simulink model "ThreeDOFsys"  (R2019a)
settings: Solver=ode3  StartTime=0.0  StopTime=120.0  FixedStep=.01  RelTol=1e-3  EnableMultiTasking=on
InitFcn:
  | % k1=25/1.5; k2=5/1.5; k3=30/1.5; k4=k3; c1=2.5; c2=.5; c3=3.5;
  | % m1=2.5; m2=2; m3=3;
  | F1 = 20; F2=0; F3=20;   % Case # 1
  | % F1 = 0; F2=0; F3=0;   % Case # 2
values from neighbouring files (symbols this model uses):
  c1 = 2.5    [MASS3.m]    (also in SMsysSIM.m = 2; three_MASS.m; two_DOF_sys_sim_ALL.m = 2)
  c2 = .5    (= 0.5)    [MASS3.m]    (also in SMsysSIM.m = 1; three_MASS.m; two_DOF_sys_sim_ALL.m = 1)
  c3 = 3.5    [MASS3.m]    (also in SMsysSIM.m = 3; three_MASS.m; two_DOF_sys_sim_ALL.m = 3)
  IC = [0;0;0;0;0;0]    [MASS3.m]    (also in three_MASS.m)
  k1 = 25    [MASS3.m]    (also in SMsysSIM.m = 90; three_MASS.m; two_DOF_sys_sim_ALL.m = 90)
  k2 = 5    [MASS3.m]    (also in SMsysSIM.m = 85; three_MASS.m; two_DOF_sys_sim_ALL.m = 85)
  k3 = 30    [MASS3.m]    (also in three_MASS.m)
  k4 = k3    (= 30)    [MASS3.m]    (also in three_MASS.m)
  m1 = 10    [DOUBLE_Pedulum_Linear_2.m]    (also in DOUBLE_Pedulum_Model_2.m; MASS3.m = 2.5; SMsysSIM.m = 5; three_MASS.m = 2.5)
  m2 = 10    [DOUBLE_Pedulum_Linear_2.m]    (also in DOUBLE_Pedulum_Model_2.m; MASS3.m = 2; SMsysSIM.m = 3; three_MASS.m = 2)
  m3 = 3    [MASS3.m]    (also in three_MASS.m)
settings Model: Creator=SLE  LastModifiedBy=sulaymon.eshkabilov
settings DataIOCC: LimitDataPoints=on  SaveFormat=Array  SignalLoggingSaveFormat=ModelDataLogs  ReturnWorkspaceOutputs=off
settings OptimizationCC: ExpressionDepthLimit=2147483647  LifeSpan=inf
settings DebuggingCC: UnderspecifiedInitializationDetection=Classic  MergeDetectMultiDrivingBlocksExec=none  SolverPrmCheckMsg=warning  FcnCallInpInsideContextMsg=warning  StateNameClashWarn=warning  SFUnexpectedBacktrackingDiag=warning  SFNoUnconditionalDefaultTransitionDiag=warning  SFExecutionAtInitializationDiag=none  ArithmeticOperatorsInVariantConditions=warning
settings HardwareCC: ProdBitPerPointer=32  ProdBitPerSizeT=32  ProdBitPerPtrDiffT=32  ProdLargestAtomicFloat=None  ProdIntDivRoundTo=Undefined  ProdEndianess=Unspecified  ProdWordSize=32  ProdHWDeviceType=32-bit Generic
settings ModelReferenceCC: PropagateSignalLabelsOutOfModel=off
settings SFSimCC: SimUseLocalCustomCode=off
settings RTWCC: GenCodeOnly=on  GenerateReport=on  TLCDebug=on  TLCAssert=on  RTWUseLocalCustomCode=off  RTWUseSimCustomCode=on  LaunchReport=on  TargetLang=C++
settings CodeAppCC: ForceParamTrailComments=on  StateflowObjectComments=on  UseSimReservedNames=on
settings GRTTargetCC: TargetLangStandard=C89/C90 (ANSI)  GeneratePreprocessorConditionals=Disable all  CombineOutputUpdateFcns=off  GRTInterface=on
settings ConfigComp: CovMetricSettings=dw  CovHtmlReporting=on  CovSaveCumulativeToWorkspaceVar=on  CovSaveSingleToWorkspaceVar=on  CovExternalEMLEnable=off

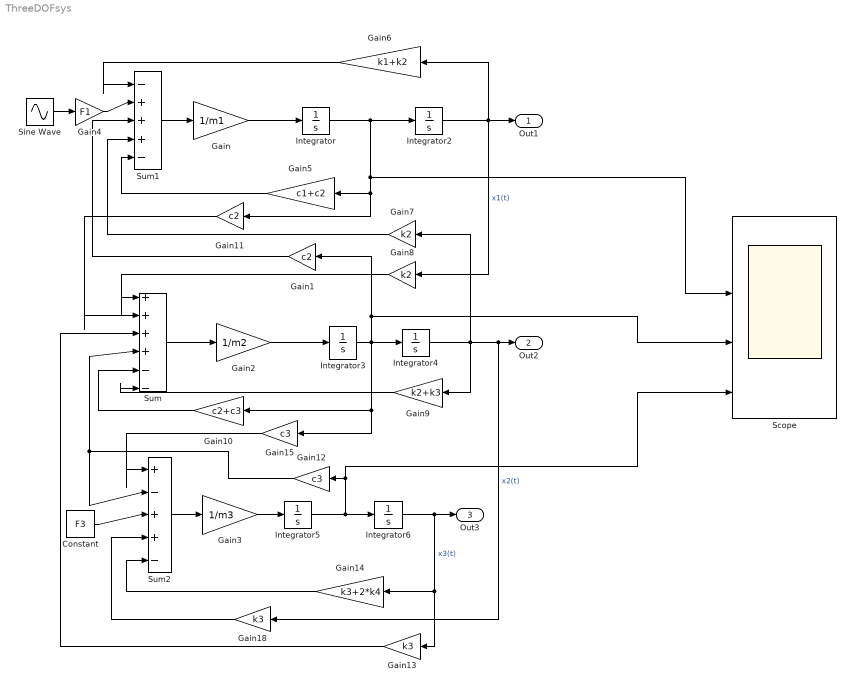
== system ThreeDOFsys ==
  Constant : Constant  Value=F3
  Gain : Gain  Gain=1/m1
  Gain1 : Gain  Gain=c2
  Gain10 : Gain  Gain=c2+c3
  Gain11 : Gain  Gain=c2
  Gain12 : Gain  Gain=c3
  Gain13 : Gain  Gain=k3
  Gain14 : Gain  Gain=k3+2*k4
  Gain15 : Gain  Gain=c3
  Gain18 : Gain  Gain=k3
  Gain2 : Gain  Gain=1/m2
  Gain3 : Gain  Gain=1/m3
  Gain4 : Gain  Gain=F1
  Gain5 : Gain  Gain=c1+c2
  Gain6 : Gain  Gain=k1+k2
  Gain7 : Gain  Gain=k2
  Gain8 : Gain  Gain=k2
  Gain9 : Gain  Gain=k2+k3
  Integrator : Integrator  InitialCondition=IC(2)
  Integrator2 : Integrator  InitialCondition=IC(1)
  Integrator3 : Integrator  InitialCondition=IC(4)
  Integrator4 : Integrator  InitialCondition=IC(3)
  Integrator5 : Integrator  InitialCondition=IC(6)
  Integrator6 : Integrator  InitialCondition=IC(5)
  Scope : Scope  NumInputPorts=4
  Sine Wave : Sin  Frequency=120  SampleTime=0
  Sum : Sum  RequirementInfo={'other' '\\192.168.1.2\sharingfiles\ENGITEC___docs\Timesheet_Dilmurod\Timesheet_en_Dilmurod_4.xls' '@Simulink_requirement_item_1' 'true' 'Preparation reading materials for Lab7 in Uzbek. Lesson 7. Assembly part. Assembly of parts (example: Internal Combustion Engine)' '' } %GIDa_704789eb_be9d_44f4_ac79_34f9d4db8dad  Inputs=|++++--
  Sum1 : Sum  Inputs=|-+++-
  Sum2 : Sum  Inputs=|+-++-
  Out1 : Outport
  Out2 : Outport  Port=2
  Out3 : Outport  Port=3
  wires:
  Gain/1 -> Integrator/1
  Integrator/1 -> Integrator2/1, Scope/2, Gain11/1, Gain5/1
  Integrator2/1 -> Out1/1, Gain6/1, Gain8/1  "x1(t)"
  Gain2/1 -> Integrator3/1
  Integrator3/1 -> Integrator4/1, Gain15/1, Gain10/1, Scope/3, Gain1/1
  Integrator4/1 -> Gain18/1, Out2/1, Gain7/1, Gain9/1  "x2(t)"
  Gain3/1 -> Integrator5/1
  Integrator5/1 -> Integrator6/1, Scope/4, Gain12/1
  Integrator6/1 -> Gain13/1, Gain14/1, Out3/1  "x3(t)"
  Sum1/1 -> Gain/1
  Sum/1 -> Gain2/1
  Sum2/1 -> Gain3/1
  Gain6/1 -> Sum1/1
  Gain5/1 -> Sum1/5
  Gain7/1 -> Sum1/4
  Gain1/1 -> Sum1/3
  Gain8/1 -> Sum/1
  Gain11/1 -> Sum/2
  Gain9/1 -> Sum/6
  Gain10/1 -> Sum/5
  Gain12/1 -> Sum/4, Sum2/2
  Gain15/1 -> Sum2/1
  Constant/1 -> Sum2/3
  Gain13/1 -> Sum/3
  Sine Wave/1 -> Gain4/1
  Gain4/1 -> Sum1/2
  Gain14/1 -> Sum2/5
  Gain18/1 -> Sum2/4
